simulink model "iiwa_IK_ROS"  (R2016b)
settings: Solver=FixedStepAuto  StartTime=0.0  StopTime=inf  FixedStep=0.05  RelTol=1e-3
model workspace (MAT data in the model file):
  SL_ROS_VariableLengthArrays_MaxSizes : struct (value not decoded)
libraries: robotlib x5
(part 2 of 3)

== matlab function iiwa_IK_ROS/IK/ik_solver ==
  data: js_cur_msg input; q_new output Bus: SL_Bus_iiwa_IK_ROS_sensor_msgs_JointState; E input; dQ output
% Based on transformation between /iiwa_base_link and /target_frame from tf
% as on error IK problem is solved and corresponding joint angles 
% changes is sent to arm_state topic

function [q_new, dQ]  = fcn(js_cur_msg, E)

persistent seq;
if isempty(seq)
    seq = 0;
end

q_new = js_cur_msg;
%n = q_new.Position_SL_Info.CurrentLength;

d01 = 0.36;
d23 = 0.42;
d45 = 0.4;
d67 = 0.126;

th1 = q_new.Position(1);
th2 = q_new.Position(2);
th3 = q_new.Position(3);
th4 = q_new.Position(4);
th5 = q_new.Position(5);
th6 = q_new.Position(6);
th7 = q_new.Position(7);

J7 = [ d67*(cos(th6)*(sin(th4)*(cos(th1)*sin(th3) + cos(th2)*cos(th3)*sin(th1)) + cos(th4)*sin(th1)*sin(th2)) + sin(th6)*(cos(th5)*(cos(th4)*(cos(th1)*sin(th3) + cos(th2)*cos(th3)*sin(th1)) - sin(th1)*sin(th2)*sin(th4)) + sin(th5)*(cos(th1)*cos(th3) - cos(th2)*sin(th1)*sin(th3)))) + d45*(sin(th4)*(cos(th1)*sin(th3) + cos(th2)*cos(th3)*sin(th1)) + cos(th4)*sin(th1)*sin(th2)) + d23*sin(th1)*sin(th2),                                                                                                                                                                                                                                                                                                                                                                                                                                                                                                                                                                                       -cos(th1)*(d45*(cos(th2)*cos(th4) - cos(th3)*sin(th2)*sin(th4)) - d67*(sin(th6)*(cos(th5)*(cos(th2)*sin(th4) + cos(th3)*cos(th4)*sin(th2)) - sin(th2)*sin(th3)*sin(th5)) - cos(th6)*(cos(th2)*cos(th4) - cos(th3)*sin(th2)*sin(th4))) + d23*cos(th2)),                                                                                                                                                                          cos(th2)*(d67*(cos(th6)*(sin(th4)*(cos(th1)*sin(th3) + cos(th2)*cos(th3)*sin(th1)) + cos(th4)*sin(th1)*sin(th2)) + sin(th6)*(cos(th5)*(cos(th4)*(cos(th1)*sin(th3) + cos(th2)*cos(th3)*sin(th1)) - sin(th1)*sin(th2)*sin(th4)) + sin(th5)*(cos(th1)*cos(th3) - cos(th2)*sin(th1)*sin(th3)))) + d45*(sin(th4)*(cos(th1)*sin(th3) + cos(th2)*cos(th3)*sin(th1)) + cos(th4)*sin(th1)*sin(th2)) + d23*sin(th1)*sin(th2)) - sin(th1)*sin(th2)*(d45*(cos(th2)*cos(th4) - cos(th3)*sin(th2)*sin(th4)) - d67*(sin(th6)*(cos(th5)*(cos(th2)*sin(th4) + cos(th3)*cos(th4)*sin(th2)) - sin(th2)*sin(th3)*sin(th5)) - cos(th6)*(cos(th2)*cos(th4) - cos(th3)*sin(th2)*sin(th4))) + d23*cos(th2)),                                                                                                                                                                                       sin(th2)*sin(th3)*(d67*(cos(th6)*(sin(th4)*(cos(th1)*sin(th3) + cos(th2)*cos(th3)*sin(th1)) + cos(th4)*sin(th1)*sin(th2)) + sin(th6)*(cos(th5)*(cos(th4)*(cos(th1)*sin(th3) + cos(th2)*cos(th3)*sin(th1)) - sin(th1)*sin(th2)*sin(th4)) + sin(th5)*(cos(th1)*cos(th3) - cos(th2)*sin(th1)*sin(th3)))) + d45*(sin(th4)*(cos(th1)*sin(th3) + cos(th2)*cos(th3)*sin(th1)) + cos(th4)*sin(th1)*sin(th2))) - (cos(th1)*cos(th3) - cos(th2)*sin(th1)*sin(th3))*(d45*(cos(th2)*cos(th4) - cos(th3)*sin(th2)*sin(th4)) - d67*(sin(th6)*(cos(th5)*(cos(th2)*sin(th4) + cos(th3)*cos(th4)*sin(th2)) - sin(th2)*sin(th3)*sin(th5)) - cos(th6)*(cos(th2)*cos(th4) - cos(th3)*sin(th2)*sin(th4)))),                                                                                                                                                                                                (cos(th2)*cos(th4) - cos(th3)*sin(th2)*sin(th4))*(d67*(cos(th6)*(sin(th4)*(cos(th1)*sin(th3) + cos(th2)*cos(th3)*sin(th1)) + cos(th4)*sin(th1)*sin(th2)) + sin(th6)*(cos(th5)*(cos(th4)*(cos(th1)*sin(th3) + cos(th2)*cos(th3)*sin(th1)) - sin(th1)*sin(th2)*sin(th4)) + sin(th5)*(cos(th1)*cos(th3) - cos(th2)*sin(th1)*sin(th3)))) + d45*(sin(th4)*(cos(th1)*sin(th3) + cos(th2)*cos(th3)*sin(th1)) + cos(th4)*sin(th1)*sin(th2))) - (sin(th4)*(cos(th1)*sin(th3) + cos(th2)*cos(th3)*sin(th1)) + cos(th4)*sin(th1)*sin(th2))*(d45*(cos(th2)*cos(th4) - cos(th3)*sin(th2)*sin(th4)) - d67*(sin(th6)*(cos(th5)*(cos(th2)*sin(th4) + cos(th3)*cos(th4)*sin(th2)) - sin(th2)*sin(th3)*sin(th5)) - cos(th6)*(cos(th2)*cos(th4) - cos(th3)*sin(th2)*sin(th4)))),                                                                                                                                                                                       d67*(sin(th5)*(cos(th2)*sin(th4) + cos(th3)*cos(th4)*sin(th2)) + cos(th5)*sin(th2)*sin(th3))*(cos(th6)*(sin(th4)*(cos(th1)*sin(th3) + cos(th2)*cos(th3)*sin(th1)) + cos(th4)*sin(th1)*sin(th2)) + sin(th6)*(cos(th5)*(cos(th4)*(cos(th1)*sin(th3) + cos(th2)*cos(th3)*sin(th1)) - sin(th1)*sin(th2)*sin(th4)) + sin(th5)*(cos(th1)*cos(th3) - cos(th2)*sin(th1)*sin(th3)))) - d67*(sin(th5)*(cos(th4)*(cos(th1)*sin(th3) + cos(th2)*cos(th3)*sin(th1)) - sin(th1)*sin(th2)*sin(th4)) - cos(th5)*(cos(th1)*cos(th3) - cos(th2)*sin(th1)*sin(th3)))*(sin(th6)*(cos(th5)*(cos(th2)*sin(th4) + cos(th3)*cos(th4)*sin(th2)) - sin(th2)*sin(th3)*sin(th5)) - cos(th6)*(cos(th2)*cos(th4) - cos(th3)*sin(th2)*sin(th4))),                                                                                                                                                                                                                                                                              0;...
 d67*(cos(th6)*(sin(th4)*(sin(th1)*sin(th3) - cos(th1)*cos(th2)*cos(th3)) - cos(th1)*cos(th4)*sin(th2)) + sin(th6)*(cos(th5)*(cos(th4)*(sin(th1)*sin(th3) - cos(th1)*cos(th2)*cos(th3)) + cos(th1)*sin(th2)*sin(th4)) + sin(th5)*(cos(th3)*sin(th1) + cos(th1)*cos(th2)*sin(th3)))) + d45*(sin(th4)*(sin(th1)*sin(th3) - cos(th1)*cos(th2)*cos(th3)) - cos(th1)*cos(th4)*sin(th2)) - d23*cos(th1)*sin(th2),                                                                                                                                                                                                                                                                                                                                                                                                                                                                                                                                                                                       -sin(th1)*(d45*(cos(th2)*cos(th4) - cos(th3)*sin(th2)*sin(th4)) - d67*(sin(th6)*(cos(th5)*(cos(th2)*sin(th4) + cos(th3)*cos(th4)*sin(th2)) - sin(th2)*sin(th3)*sin(th5)) - cos(th6)*(cos(th2)*cos(th4) - cos(th3)*sin(th2)*sin(th4))) + d23*cos(th2)),                                                                                                                                                                          cos(th2)*(d67*(cos(th6)*(sin(th4)*(sin(th1)*sin(th3) - cos(th1)*cos(th2)*cos(th3)) - cos(th1)*cos(th4)*sin(th2)) + sin(th6)*(cos(th5)*(cos(th4)*(sin(th1)*sin(th3) - cos(th1)*cos(th2)*cos(th3)) + cos(th1)*sin(th2)*sin(th4)) + sin(th5)*(cos(th3)*sin(th1) + cos(th1)*cos(th2)*sin(th3)))) + d45*(sin(th4)*(sin(th1)*sin(th3) - cos(th1)*cos(th2)*cos(th3)) - cos(th1)*cos(th4)*sin(th2)) - d23*cos(th1)*sin(th2)) + cos(th1)*sin(th2)*(d45*(cos(th2)*cos(th4) - cos(th3)*sin(th2)*sin(th4)) - d67*(sin(th6)*(cos(th5)*(cos(th2)*sin(th4) + cos(th3)*cos(th4)*sin(th2)) - sin(th2)*sin(th3)*sin(th5)) - cos(th6)*(cos(th2)*cos(th4) - cos(th3)*sin(th2)*sin(th4))) + d23*cos(th2)),                                                                                                                                                                                       sin(th2)*sin(th3)*(d67*(cos(th6)*(sin(th4)*(sin(th1)*sin(th3) - cos(th1)*cos(th2)*cos(th3)) - cos(th1)*cos(th4)*sin(th2)) + sin(th6)*(cos(th5)*(cos(th4)*(sin(th1)*sin(th3) - cos(th1)*cos(th2)*cos(th3)) + cos(th1)*sin(th2)*sin(th4)) + sin(th5)*(cos(th3)*sin(th1) + cos(th1)*cos(th2)*sin(th3)))) + d45*(sin(th4)*(sin(th1)*sin(th3) - cos(th1)*cos(th2)*cos(th3)) - cos(th1)*cos(th4)*sin(th2))) - (cos(th3)*sin(th1) + cos(th1)*cos(th2)*sin(th3))*(d45*(cos(th2)*cos(th4) - cos(th3)*sin(th2)*sin(th4)) - d67*(sin(th6)*(cos(th5)*(cos(th2)*sin(th4) + cos(th3)*cos(th4)*sin(th2)) - sin(th2)*sin(th3)*sin(th5)) - cos(th6)*(cos(th2)*cos(th4) - cos(th3)*sin(th2)*sin(th4)))),                                                                                                                                                                                                (d67*(cos(th6)*(sin(th4)*(sin(th1)*sin(th3) - cos(th1)*cos(th2)*cos(th3)) - cos(th1)*cos(th4)*sin(th2)) + sin(th6)*(cos(th5)*(cos(th4)*(sin(th1)*sin(th3) - cos(th1)*cos(th2)*cos(th3)) + cos(th1)*sin(th2)*sin(th4)) + sin(th5)*(cos(th3)*sin(th1) + cos(th1)*cos(th2)*sin(th3)))) + d45*(sin(th4)*(sin(th1)*sin(th3) - cos(th1)*cos(th2)*cos(th3)) - cos(th1)*cos(th4)*sin(th2)))*(cos(th2)*cos(th4) - cos(th3)*sin(th2)*sin(th4)) - (sin(th4)*(sin(th1)*sin(th3) - cos(th1)*cos(th2)*cos(th3)) - cos(th1)*cos(th4)*sin(th2))*(d45*(cos(th2)*cos(th4) - cos(th3)*sin(th2)*sin(th4)) - d67*(sin(th6)*(cos(th5)*(cos(th2)*sin(th4) + cos(th3)*cos(th4)*sin(th2)) - sin(th2)*sin(th3)*sin(th5)) - cos(th6)*(cos(th2)*cos(th4) - cos(th3)*sin(th2)*sin(th4)))),                                                                                                                                                                                       d67*(sin(th5)*(cos(th2)*sin(th4) + cos(th3)*cos(th4)*sin(th2)) + cos(th5)*sin(th2)*sin(th3))*(cos(th6)*(sin(th4)*(sin(th1)*sin(th3) - cos(th1)*cos(th2)*cos(th3)) - cos(th1)*cos(th4)*sin(th2)) + sin(th6)*(cos(th5)*(cos(th4)*(sin(th1)*sin(th3) - cos(th1)*cos(th2)*cos(th3)) + cos(th1)*sin(th2)*sin(th4)) + sin(th5)*(cos(th3)*sin(th1) + cos(th1)*cos(th2)*sin(th3)))) - d67*(sin(th5)*(cos(th4)*(sin(th1)*sin(th3) - cos(th1)*cos(th2)*cos(th3)) + cos(th1)*sin(th2)*sin(th4)) - cos(th5)*(cos(th3)*sin(th1) + cos(th1)*cos(th2)*sin(th3)))*(sin(th6)*(cos(th5)*(cos(th2)*sin(th4) + cos(th3)*cos(th4)*sin(th2)) - sin(th2)*sin(th3)*sin(th5)) - cos(th6)*(cos(th2)*cos(th4) - cos(th3)*sin(th2)*sin(th4))),                                                                                                                                                                                                                                                                              0;...
                                                                                                                                                                                                                                                                                                                                                                                                         0, cos(th1)*(d67*(cos(th6)*(sin(th4)*(sin(th1)*sin(th3) - cos(th1)*cos(th2)*cos(th3)) - cos(th1)*cos(th4)*sin(th2)) + sin(th6)*(cos(th5)*(cos(th4)*(sin(th1)*sin(th3) - cos(th1)*cos(th2)*cos(th3)) + cos(th1)*sin(th2)*sin(th4)) + sin(th5)*(cos(th3)*sin(th1) + cos(th1)*cos(th2)*sin(th3)))) + d45*(sin(th4)*(sin(th1)*sin(th3) - cos(th1)*cos(th2)*cos(th3)) - cos(th1)*cos(th4)*sin(th2)) - d23*cos(th1)*sin(th2)) - sin(th1)*(d67*(cos(th6)*(sin(th4)*(cos(th1)*sin(th3) + cos(th2)*cos(th3)*sin(th1)) + cos(th4)*sin(th1)*sin(th2)) + sin(th6)*(cos(th5)*(cos(th4)*(cos(th1)*sin(th3) + cos(th2)*cos(th3)*sin(th1)) - sin(th1)*sin(th2)*sin(th4)) + sin(th5)*(cos(th1)*cos(th3) - cos(th2)*sin(th1)*sin(th3)))) + d45*(sin(th4)*(cos(th1)*sin(th3) + cos(th2)*cos(th3)*sin(th1)) + cos(th4)*sin(th1)*sin(th2)) + d23*sin(th1)*sin(th2)), sin(th1)*sin(th2)*(d67*(cos(th6)*(sin(th4)*(sin(th1)*sin(th3) - cos(th1)*cos(th2)*cos(th3)) - cos(th1)*cos(th4)*sin(th2)) + sin(th6)*(cos(th5)*(cos(th4)*(sin(th1)*sin(th3) - cos(th1)*cos(th2)*cos(th3)) + cos(th1)*sin(th2)*sin(th4)) + sin(th5)*(cos(th3)*sin(th1) + cos(th1)*cos(th2)*sin(th3)))) + d45*(sin(th4)*(sin(th1)*sin(th3) - cos(th1)*cos(th2)*cos(th3)) - cos(th1)*cos(th4)*sin(th2)) - d23*cos(th1)*sin(th2)) + cos(th1)*sin(th2)*(d67*(cos(th6)*(sin(th4)*(cos(th1)*sin(th3) + cos(th2)*cos(th3)*sin(th1)) + cos(th4)*sin(th1)*sin(th2)) + sin(th6)*(cos(th5)*(cos(th4)*(cos(th1)*sin(th3) + cos(th2)*cos(th3)*sin(th1)) - sin(th1)*sin(th2)*sin(th4)) + sin(th5)*(cos(th1)*cos(th3) - cos(th2)*sin(th1)*sin(th3)))) + d45*(sin(th4)*(cos(th1)*sin(th3) + cos(th2)*cos(th3)*sin(th1)) + cos(th4)*sin(th1)*sin(th2)) + d23*sin(th1)*sin(th2)), (d67*(cos(th6)*(sin(th4)*(sin(th1)*sin(th3) - cos(th1)*cos(th2)*cos(th3)) - cos(th1)*cos(th4)*sin(th2)) + sin(th6)*(cos(th5)*(cos(th4)*(sin(th1)*sin(th3) - cos(th1)*cos(th2)*cos(th3)) + cos(th1)*sin(th2)*sin(th4)) + sin(th5)*(cos(th3)*sin(th1) + cos(th1)*cos(th2)*sin(th3)))) + d45*(sin(th4)*(sin(th1)*sin(th3) - cos(th1)*cos(th2)*cos(th3)) - cos(th1)*cos(th4)*sin(th2)))*(cos(th1)*cos(th3) - cos(th2)*sin(th1)*sin(th3)) - (cos(th3)*sin(th1) + cos(th1)*cos(th2)*sin(th3))*(d67*(cos(th6)*(sin(th4)*(cos(th1)*sin(th3) + cos(th2)*cos(th3)*sin(th1)) + cos(th4)*sin(th1)*sin(th2)) + sin(th6)*(cos(th5)*(cos(th4)*(cos(th1)*sin(th3) + cos(th2)*cos(th3)*sin(th1)) - sin(th1)*sin(th2)*sin(th4)) + sin(th5)*(cos(th1)*cos(th3) - cos(th2)*sin(th1)*sin(th3)))) + d45*(sin(th4)*(cos(th1)*sin(th3) + cos(th2)*cos(th3)*sin(th1)) + cos(th4)*sin(th1)*sin(th2))), (sin(th4)*(cos(th1)*sin(th3) + cos(th2)*cos(th3)*sin(th1)) + cos(th4)*sin(th1)*sin(th2))*(d67*(cos(th6)*(sin(th4)*(sin(th1)*sin(th3) - cos(th1)*cos(th2)*cos(th3)) - cos(th1)*cos(th4)*sin(th2)) + sin(th6)*(cos(th5)*(cos(th4)*(sin(th1)*sin(th3) - cos(th1)*cos(th2)*cos(th3)) + cos(th1)*sin(th2)*sin(th4)) + sin(th5)*(cos(th3)*sin(th1) + cos(th1)*cos(th2)*sin(th3)))) + d45*(sin(th4)*(sin(th1)*sin(th3) - cos(th1)*cos(th2)*cos(th3)) - cos(th1)*cos(th4)*sin(th2))) - (sin(th4)*(sin(th1)*sin(th3) - cos(th1)*cos(th2)*cos(th3)) - cos(th1)*cos(th4)*sin(th2))*(d67*(cos(th6)*(sin(th4)*(cos(th1)*sin(th3) + cos(th2)*cos(th3)*sin(th1)) + cos(th4)*sin(th1)*sin(th2)) + sin(th6)*(cos(th5)*(cos(th4)*(cos(th1)*sin(th3) + cos(th2)*cos(th3)*sin(th1)) - sin(th1)*sin(th2)*sin(th4)) + sin(th5)*(cos(th1)*cos(th3) - cos(th2)*sin(th1)*sin(th3)))) + d45*(sin(th4)*(cos(th1)*sin(th3) + cos(th2)*cos(th3)*sin(th1)) + cos(th4)*sin(th1)*sin(th2))), d67*(sin(th5)*(cos(th4)*(sin(th1)*sin(th3) - cos(th1)*cos(th2)*cos(th3)) + cos(th1)*sin(th2)*sin(th4)) - cos(th5)*(cos(th3)*sin(th1) + cos(th1)*cos(th2)*sin(th3)))*(cos(th6)*(sin(th4)*(cos(th1)*sin(th3) + cos(th2)*cos(th3)*sin(th1)) + cos(th4)*sin(th1)*sin(th2)) + sin(th6)*(cos(th5)*(cos(th4)*(cos(th1)*sin(th3) + cos(th2)*cos(th3)*sin(th1)) - sin(th1)*sin(th2)*sin(th4)) + sin(th5)*(cos(th1)*cos(th3) - cos(th2)*sin(th1)*sin(th3)))) - d67*(cos(th6)*(sin(th4)*(sin(th1)*sin(th3) - cos(th1)*cos(th2)*cos(th3)) - cos(th1)*cos(th4)*sin(th2)) + sin(th6)*(cos(th5)*(cos(th4)*(sin(th1)*sin(th3) - cos(th1)*cos(th2)*cos(th3)) + cos(th1)*sin(th2)*sin(th4)) + sin(th5)*(cos(th3)*sin(th1) + cos(th1)*cos(th2)*sin(th3))))*(sin(th5)*(cos(th4)*(cos(th1)*sin(th3) + cos(th2)*cos(th3)*sin(th1)) - sin(th1)*sin(th2)*sin(th4)) - cos(th5)*(cos(th1)*cos(th3) - cos(th2)*sin(th1)*sin(th3))),                                                                                                                                                                                                                                                                              0;...
                                                                                                                                                                                                                                                                                                                                                                                                         0,                                                                                                                                                                                                                                                                                                                                                                                                                                                                                                                                                                                                                                                                                                                                                                                                                                    sin(th1),                                                                                                                                                                                                                                                                                                                                                                                                                                                                                                                                                                                                                                                                                                                                                                                                                                            -cos(th1)*sin(th2),                                                                                                                                                                                                                                                                                                                                                                                                                                                                                                                                                                                                                                                                                                                                                                                                                              cos(th3)*sin(th1) + cos(th1)*cos(th2)*sin(th3),                                                                                                                                                                                                                                                                                                                                                                                                                                                                                                                                                                                                                                                                                                                                                                                                                                                                      sin(th4)*(sin(th1)*sin(th3) - cos(th1)*cos(th2)*cos(th3)) - cos(th1)*cos(th4)*sin(th2),                                                                                                                                                                                                                                                                                                                                                                                                                                                                                                                                                                                                                                                                                                                                           cos(th5)*(cos(th3)*sin(th1) + cos(th1)*cos(th2)*sin(th3)) - sin(th5)*(cos(th4)*(sin(th1)*sin(th3) - cos(th1)*cos(th2)*cos(th3)) + cos(th1)*sin(th2)*sin(th4)),   cos(th6)*(sin(th4)*(sin(th1)*sin(th3) - cos(th1)*cos(th2)*cos(th3)) - cos(th1)*cos(th4)*sin(th2)) + sin(th6)*(cos(th5)*(cos(th4)*(sin(th1)*sin(th3) - cos(th1)*cos(th2)*cos(th3)) + cos(th1)*sin(th2)*sin(th4)) + sin(th5)*(cos(th3)*sin(th1) + cos(th1)*cos(th2)*sin(th3)));...
                                                                                                                                                                                                                                                                                                                                                                                                         0,                                                                                                                                                                                                                                                                                                                                                                                                                                                                                                                                                                                                                                                                                                                                                                                                                                   -cos(th1),                                                                                                                                                                                                                                                                                                                                                                                                                                                                                                                                                                                                                                                                                                                                                                                                                                            -sin(th1)*sin(th2),                                                                                                                                                                                                                                                                                                                                                                                                                                                                                                                                                                                                                                                                                                                                                                                                                              cos(th2)*sin(th1)*sin(th3) - cos(th1)*cos(th3),                                                                                                                                                                                                                                                                                                                                                                                                                                                                                                                                                                                                                                                                                                                                                                                                                                                                    - sin(th4)*(cos(th1)*sin(th3) + cos(th2)*cos(th3)*sin(th1)) - cos(th4)*sin(th1)*sin(th2),                                                                                                                                                                                                                                                                                                                                                                                                                                                                                                                                                                                                                                                                                                                                           sin(th5)*(cos(th4)*(cos(th1)*sin(th3) + cos(th2)*cos(th3)*sin(th1)) - sin(th1)*sin(th2)*sin(th4)) - cos(th5)*(cos(th1)*cos(th3) - cos(th2)*sin(th1)*sin(th3)), - cos(th6)*(sin(th4)*(cos(th1)*sin(th3) + cos(th2)*cos(th3)*sin(th1)) + cos(th4)*sin(th1)*sin(th2)) - sin(th6)*(cos(th5)*(cos(th4)*(cos(th1)*sin(th3) + cos(th2)*cos(th3)*sin(th1)) - sin(th1)*sin(th2)*sin(th4)) + sin(th5)*(cos(th1)*cos(th3) - cos(th2)*sin(th1)*sin(th3)));...
                                                                                                                                                                                                                                                                                                                                                                                                         1,                                                                                                                                                                                                                                                                                                                                                                                                                                                                                                                                                                                                                                                                                                                                                                                                                                           0,                                                                                                                                                                                                                                                                                                                                                                                                                                                                                                                                                                                                                                                                                                                                                                                                                                                      cos(th2),                                                                                                                                                                                                                                                                                                                                                                                                                                                                                                                                                                                                                                                                                                                                                                                                                                                           sin(th2)*sin(th3),                                                                                                                                                                                                                                                                                                                                                                                                                                                                                                                                                                                                                                                                                                                                                                                                                                                                                                              cos(th2)*cos(th4) - cos(th3)*sin(th2)*sin(th4),                                                                                                                                                                                                                                                                                                                                                                                                                                                                                                                                                                                                                                                                                                                                                                                                                  sin(th5)*(cos(th2)*sin(th4) + cos(th3)*cos(th4)*sin(th2)) + cos(th5)*sin(th2)*sin(th3),                                                                                                                  cos(th6)*(cos(th2)*cos(th4) - cos(th3)*sin(th2)*sin(th4)) - sin(th6)*(cos(th5)*(cos(th2)*sin(th4) + cos(th3)*cos(th4)*sin(th2)) - sin(th2)*sin(th3)*sin(th5))];
%%%%%%%%%%%%%%%%%%%%%%%%%%%%%%%%%%%%%%%%%%%%%

J7t = [                                                                                                                                                                                                                                                                                                                                                    d67*(cos(th6)*(sin(th4)*(cos(th1)*sin(th3) + cos(th2)*cos(th3)*sin(th1)) + cos(th4)*sin(th1)*sin(th2)) + sin(th6)*(cos(th5)*(cos(th4)*(cos(th1)*sin(th3) + cos(th2)*cos(th3)*sin(th1)) - sin(th1)*sin(th2)*sin(th4)) + sin(th5)*(cos(th1)*cos(th3) - cos(th2)*sin(th1)*sin(th3)))) + d45*(sin(th4)*(cos(th1)*sin(th3) + cos(th2)*cos(th3)*sin(th1)) + cos(th4)*sin(th1)*sin(th2)) + d23*sin(th1)*sin(th2),                                                                                                                                                                                                                                                                                                                                                    d67*(cos(th6)*(sin(th4)*(sin(th1)*sin(th3) - cos(th1)*cos(th2)*cos(th3)) - cos(th1)*cos(th4)*sin(th2)) + sin(th6)*(cos(th5)*(cos(th4)*(sin(th1)*sin(th3) - cos(th1)*cos(th2)*cos(th3)) + cos(th1)*sin(th2)*sin(th4)) + sin(th5)*(cos(th3)*sin(th1) + cos(th1)*cos(th2)*sin(th3)))) + d45*(sin(th4)*(sin(th1)*sin(th3) - cos(th1)*cos(th2)*cos(th3)) - cos(th1)*cos(th4)*sin(th2)) - d23*cos(th1)*sin(th2),                                                                                                                                                                                                                                                                                                                                                                                                                                                                                                                                                                                                                                                                                                                                                                                                                                                                                                                                                           0,                                                                                                                                                                                                                                                                            0,                                                                                                                                                                                                                                                                              0,                                                                                                                                                             1;...
                                                                                                                                                                                                                                                                                                                                                                                                                                                                                                        -cos(th1)*(d45*(cos(th2)*cos(th4) - cos(th3)*sin(th2)*sin(th4)) - d67*(sin(th6)*(cos(th5)*(cos(th2)*sin(th4) + cos(th3)*cos(th4)*sin(th2)) - sin(th2)*sin(th3)*sin(th5)) - cos(th6)*(cos(th2)*cos(th4) - cos(th3)*sin(th2)*sin(th4))) + d23*cos(th2)),                                                                                                                                                                                                                                                                                                                                                                                                                                                                                                        -sin(th1)*(d45*(cos(th2)*cos(th4) - cos(th3)*sin(th2)*sin(th4)) - d67*(sin(th6)*(cos(th5)*(cos(th2)*sin(th4) + cos(th3)*cos(th4)*sin(th2)) - sin(th2)*sin(th3)*sin(th5)) - cos(th6)*(cos(th2)*cos(th4) - cos(th3)*sin(th2)*sin(th4))) + d23*cos(th2)),                                                                                                                 cos(th1)*(d67*(cos(th6)*(sin(th4)*(sin(th1)*sin(th3) - cos(th1)*cos(th2)*cos(th3)) - cos(th1)*cos(th4)*sin(th2)) + sin(th6)*(cos(th5)*(cos(th4)*(sin(th1)*sin(th3) - cos(th1)*cos(th2)*cos(th3)) + cos(th1)*sin(th2)*sin(th4)) + sin(th5)*(cos(th3)*sin(th1) + cos(th1)*cos(th2)*sin(th3)))) + d45*(sin(th4)*(sin(th1)*sin(th3) - cos(th1)*cos(th2)*cos(th3)) - cos(th1)*cos(th4)*sin(th2)) - d23*cos(th1)*sin(th2)) - sin(th1)*(d67*(cos(th6)*(sin(th4)*(cos(th1)*sin(th3) + cos(th2)*cos(th3)*sin(th1)) + cos(th4)*sin(th1)*sin(th2)) + sin(th6)*(cos(th5)*(cos(th4)*(cos(th1)*sin(th3) + cos(th2)*cos(th3)*sin(th1)) - sin(th1)*sin(th2)*sin(th4)) + sin(th5)*(cos(th1)*cos(th3) - cos(th2)*sin(th1)*sin(th3)))) + d45*(sin(th4)*(cos(th1)*sin(th3) + cos(th2)*cos(th3)*sin(th1)) + cos(th4)*sin(th1)*sin(th2)) + d23*sin(th1)*sin(th2)),                                                                                                                                                                                                                                                                     sin(th1),                                                                                                                                                                                                                                                                      -cos(th1),                                                                                                                                                             0;...
                                                                         cos(th2)*(d67*(cos(th6)*(sin(th4)*(cos(th1)*sin(th3) + cos(th2)*cos(th3)*sin(th1)) + cos(th4)*sin(th1)*sin(th2)) + sin(th6)*(cos(th5)*(cos(th4)*(cos(th1)*sin(th3) + cos(th2)*cos(th3)*sin(th1)) - sin(th1)*sin(th2)*sin(th4)) + sin(th5)*(cos(th1)*cos(th3) - cos(th2)*sin(th1)*sin(th3)))) + d45*(sin(th4)*(cos(th1)*sin(th3) + cos(th2)*cos(th3)*sin(th1)) + cos(th4)*sin(th1)*sin(th2)) + d23*sin(th1)*sin(th2)) - sin(th1)*sin(th2)*(d45*(cos(th2)*cos(th4) - cos(th3)*sin(th2)*sin(th4)) - d67*(sin(th6)*(cos(th5)*(cos(th2)*sin(th4) + cos(th3)*cos(th4)*sin(th2)) - sin(th2)*sin(th3)*sin(th5)) - cos(th6)*(cos(th2)*cos(th4) - cos(th3)*sin(th2)*sin(th4))) + d23*cos(th2)),                                                                         cos(th2)*(d67*(cos(th6)*(sin(th4)*(sin(th1)*sin(th3) - cos(th1)*cos(th2)*cos(th3)) - cos(th1)*cos(th4)*sin(th2)) + sin(th6)*(cos(th5)*(cos(th4)*(sin(th1)*sin(th3) - cos(th1)*cos(th2)*cos(th3)) + cos(th1)*sin(th2)*sin(th4)) + sin(th5)*(cos(th3)*sin(th1) + cos(th1)*cos(th2)*sin(th3)))) + d45*(sin(th4)*(sin(th1)*sin(th3) - cos(th1)*cos(th2)*cos(th3)) - cos(th1)*cos(th4)*sin(th2)) - d23*cos(th1)*sin(th2)) + cos(th1)*sin(th2)*(d45*(cos(th2)*cos(th4) - cos(th3)*sin(th2)*sin(th4)) - d67*(sin(th6)*(cos(th5)*(cos(th2)*sin(th4) + cos(th3)*cos(th4)*sin(th2)) - sin(th2)*sin(th3)*sin(th5)) - cos(th6)*(cos(th2)*cos(th4) - cos(th3)*sin(th2)*sin(th4))) + d23*cos(th2)),                                                                                               sin(th1)*sin(th2)*(d67*(cos(th6)*(sin(th4)*(sin(th1)*sin(th3) - cos(th1)*cos(th2)*cos(th3)) - cos(th1)*cos(th4)*sin(th2)) + sin(th6)*(cos(th5)*(cos(th4)*(sin(th1)*sin(th3) - cos(th1)*cos(th2)*cos(th3)) + cos(th1)*sin(th2)*sin(th4)) + sin(th5)*(cos(th3)*sin(th1) + cos(th1)*cos(th2)*sin(th3)))) + d45*(sin(th4)*(sin(th1)*sin(th3) - cos(th1)*cos(th2)*cos(th3)) - cos(th1)*cos(th4)*sin(th2)) - d23*cos(th1)*sin(th2)) + cos(th1)*sin(th2)*(d67*(cos(th6)*(sin(th4)*(cos(th1)*sin(th3) + cos(th2)*cos(th3)*sin(th1)) + cos(th4)*sin(th1)*sin(th2)) + sin(th6)*(cos(th5)*(cos(th4)*(cos(th1)*sin(th3) + cos(th2)*cos(th3)*sin(th1)) - sin(th1)*sin(th2)*sin(th4)) + sin(th5)*(cos(th1)*cos(th3) - cos(th2)*sin(th1)*sin(th3)))) + d45*(sin(th4)*(cos(th1)*sin(th3) + cos(th2)*cos(th3)*sin(th1)) + cos(th4)*sin(th1)*sin(th2)) + d23*sin(th1)*sin(th2)),                                                                                                                                                                                                                                                           -cos(th1)*sin(th2),                                                                                                                                                                                                                                                             -sin(th1)*sin(th2),                                                                                                                                                      cos(th2);...
                                                                        sin(th2)*sin(th3)*(d67*(cos(th6)*(sin(th4)*(cos(th1)*sin(th3) + cos(th2)*cos(th3)*sin(th1)) + cos(th4)*sin(th1)*sin(th2)) + sin(th6)*(cos(th5)*(cos(th4)*(cos(th1)*sin(th3) + cos(th2)*cos(th3)*sin(th1)) - sin(th1)*sin(th2)*sin(th4)) + sin(th5)*(cos(th1)*cos(th3) - cos(th2)*sin(th1)*sin(th3)))) + d45*(sin(th4)*(cos(th1)*sin(th3) + cos(th2)*cos(th3)*sin(th1)) + cos(th4)*sin(th1)*sin(th2))) - (cos(th1)*cos(th3) - cos(th2)*sin(th1)*sin(th3))*(d45*(cos(th2)*cos(th4) - cos(th3)*sin(th2)*sin(th4)) - d67*(sin(th6)*(cos(th5)*(cos(th2)*sin(th4) + cos(th3)*cos(th4)*sin(th2)) - sin(th2)*sin(th3)*sin(th5)) - cos(th6)*(cos(th2)*cos(th4) - cos(th3)*sin(th2)*sin(th4)))),                                                                        sin(th2)*sin(th3)*(d67*(cos(th6)*(sin(th4)*(sin(th1)*sin(th3) - cos(th1)*cos(th2)*cos(th3)) - cos(th1)*cos(th4)*sin(th2)) + sin(th6)*(cos(th5)*(cos(th4)*(sin(th1)*sin(th3) - cos(th1)*cos(th2)*cos(th3)) + cos(th1)*sin(th2)*sin(th4)) + sin(th5)*(cos(th3)*sin(th1) + cos(th1)*cos(th2)*sin(th3)))) + d45*(sin(th4)*(sin(th1)*sin(th3) - cos(th1)*cos(th2)*cos(th3)) - cos(th1)*cos(th4)*sin(th2))) - (cos(th3)*sin(th1) + cos(th1)*cos(th2)*sin(th3))*(d45*(cos(th2)*cos(th4) - cos(th3)*sin(th2)*sin(th4)) - d67*(sin(th6)*(cos(th5)*(cos(th2)*sin(th4) + cos(th3)*cos(th4)*sin(th2)) - sin(th2)*sin(th3)*sin(th5)) - cos(th6)*(cos(th2)*cos(th4) - cos(th3)*sin(th2)*sin(th4)))),                                                                                 (d67*(cos(th6)*(sin(th4)*(sin(th1)*sin(th3) - cos(th1)*cos(th2)*cos(th3)) - cos(th1)*cos(th4)*sin(th2)) + sin(th6)*(cos(th5)*(cos(th4)*(sin(th1)*sin(th3) - cos(th1)*cos(th2)*cos(th3)) + cos(th1)*sin(th2)*sin(th4)) + sin(th5)*(cos(th3)*sin(th1) + cos(th1)*cos(th2)*sin(th3)))) + d45*(sin(th4)*(sin(th1)*sin(th3) - cos(th1)*cos(th2)*cos(th3)) - cos(th1)*cos(th4)*sin(th2)))*(cos(th1)*cos(th3) - cos(th2)*sin(th1)*sin(th3)) - (cos(th3)*sin(th1) + cos(th1)*cos(th2)*sin(th3))*(d67*(cos(th6)*(sin(th4)*(cos(th1)*sin(th3) + cos(th2)*cos(th3)*sin(th1)) + cos(th4)*sin(th1)*sin(th2)) + sin(th6)*(cos(th5)*(cos(th4)*(cos(th1)*sin(th3) + cos(th2)*cos(th3)*sin(th1)) - sin(th1)*sin(th2)*sin(th4)) + sin(th5)*(cos(th1)*cos(th3) - cos(th2)*sin(th1)*sin(th3)))) + d45*(sin(th4)*(cos(th1)*sin(th3) + cos(th2)*cos(th3)*sin(th1)) + cos(th4)*sin(th1)*sin(th2))),                                                                                                                                                                                                                               cos(th3)*sin(th1) + cos(th1)*cos(th2)*sin(th3),                                                                                                                                                                                                                                 cos(th2)*sin(th1)*sin(th3) - cos(th1)*cos(th3),                                                                                                                                             sin(th2)*sin(th3);...
 (cos(th2)*cos(th4) - cos(th3)*sin(th2)*sin(th4))*(d67*(cos(th6)*(sin(th4)*(cos(th1)*sin(th3) + cos(th2)*cos(th3)*sin(th1)) + cos(th4)*sin(th1)*sin(th2)) + sin(th6)*(cos(th5)*(cos(th4)*(cos(th1)*sin(th3) + cos(th2)*cos(th3)*sin(th1)) - sin(th1)*sin(th2)*sin(th4)) + sin(th5)*(cos(th1)*cos(th3) - cos(th2)*sin(th1)*sin(th3)))) + d45*(sin(th4)*(cos(th1)*sin(th3) + cos(th2)*cos(th3)*sin(th1)) + cos(th4)*sin(th1)*sin(th2))) - (sin(th4)*(cos(th1)*sin(th3) + cos(th2)*cos(th3)*sin(th1)) + cos(th4)*sin(th1)*sin(th2))*(d45*(cos(th2)*cos(th4) - cos(th3)*sin(th2)*sin(th4)) - d67*(sin(th6)*(cos(th5)*(cos(th2)*sin(th4) + cos(th3)*cos(th4)*sin(th2)) - sin(th2)*sin(th3)*sin(th5)) - cos(th6)*(cos(th2)*cos(th4) - cos(th3)*sin(th2)*sin(th4)))), (d67*(cos(th6)*(sin(th4)*(sin(th1)*sin(th3) - cos(th1)*cos(th2)*cos(th3)) - cos(th1)*cos(th4)*sin(th2)) + sin(th6)*(cos(th5)*(cos(th4)*(sin(th1)*sin(th3) - cos(th1)*cos(th2)*cos(th3)) + cos(th1)*sin(th2)*sin(th4)) + sin(th5)*(cos(th3)*sin(th1) + cos(th1)*cos(th2)*sin(th3)))) + d45*(sin(th4)*(sin(th1)*sin(th3) - cos(th1)*cos(th2)*cos(th3)) - cos(th1)*cos(th4)*sin(th2)))*(cos(th2)*cos(th4) - cos(th3)*sin(th2)*sin(th4)) - (sin(th4)*(sin(th1)*sin(th3) - cos(th1)*cos(th2)*cos(th3)) - cos(th1)*cos(th4)*sin(th2))*(d45*(cos(th2)*cos(th4) - cos(th3)*sin(th2)*sin(th4)) - d67*(sin(th6)*(cos(th5)*(cos(th2)*sin(th4) + cos(th3)*cos(th4)*sin(th2)) - sin(th2)*sin(th3)*sin(th5)) - cos(th6)*(cos(th2)*cos(th4) - cos(th3)*sin(th2)*sin(th4)))), (sin(th4)*(cos(th1)*sin(th3) + cos(th2)*cos(th3)*sin(th1)) + cos(th4)*sin(th1)*sin(th2))*(d67*(cos(th6)*(sin(th4)*(sin(th1)*sin(th3) - cos(th1)*cos(th2)*cos(th3)) - cos(th1)*cos(th4)*sin(th2)) + sin(th6)*(cos(th5)*(cos(th4)*(sin(th1)*sin(th3) - cos(th1)*cos(th2)*cos(th3)) + cos(th1)*sin(th2)*sin(th4)) + sin(th5)*(cos(th3)*sin(th1) + cos(th1)*cos(th2)*sin(th3)))) + d45*(sin(th4)*(sin(th1)*sin(th3) - cos(th1)*cos(th2)*cos(th3)) - cos(th1)*cos(th4)*sin(th2))) - (sin(th4)*(sin(th1)*sin(th3) - cos(th1)*cos(th2)*cos(th3)) - cos(th1)*cos(th4)*sin(th2))*(d67*(cos(th6)*(sin(th4)*(cos(th1)*sin(th3) + cos(th2)*cos(th3)*sin(th1)) + cos(th4)*sin(th1)*sin(th2)) + sin(th6)*(cos(th5)*(cos(th4)*(cos(th1)*sin(th3) + cos(th2)*cos(th3)*sin(th1)) - sin(th1)*sin(th2)*sin(th4)) + sin(th5)*(cos(th1)*cos(th3) - cos(th2)*sin(th1)*sin(th3)))) + d45*(sin(th4)*(cos(th1)*sin(th3) + cos(th2)*cos(th3)*sin(th1)) + cos(th4)*sin(th1)*sin(th2))),                                                                                                                                                                                       sin(th4)*(sin(th1)*sin(th3) - cos(th1)*cos(th2)*cos(th3)) - cos(th1)*cos(th4)*sin(th2),                                                                                                                                                                                       - sin(th4)*(cos(th1)*sin(th3) + cos(th2)*cos(th3)*sin(th1)) - cos(th4)*sin(th1)*sin(th2),                                                                                                                cos(th2)*cos(th4) - cos(th3)*sin(th2)*sin(th4);...
                                            d67*(sin(th5)*(cos(th2)*sin(th4) + cos(th3)*cos(th4)*sin(th2)) + cos(th5)*sin(th2)*sin(th3))*(cos(th6)*(sin(th4)*(cos(th1)*sin(th3) + cos(th2)*cos(th3)*sin(th1)) + cos(th4)*sin(th1)*sin(th2)) + sin(th6)*(cos(th5)*(cos(th4)*(cos(th1)*sin(th3) + cos(th2)*cos(th3)*sin(th1)) - sin(th1)*sin(th2)*sin(th4)) + sin(th5)*(cos(th1)*cos(th3) - cos(th2)*sin(th1)*sin(th3)))) - d67*(sin(th5)*(cos(th4)*(cos(th1)*sin(th3) + cos(th2)*cos(th3)*sin(th1)) - sin(th1)*sin(th2)*sin(th4)) - cos(th5)*(cos(th1)*cos(th3) - cos(th2)*sin(th1)*sin(th3)))*(sin(th6)*(cos(th5)*(cos(th2)*sin(th4) + cos(th3)*cos(th4)*sin(th2)) - sin(th2)*sin(th3)*sin(th5)) - cos(th6)*(cos(th2)*cos(th4) - cos(th3)*sin(th2)*sin(th4))),                                            d67*(sin(th5)*(cos(th2)*sin(th4) + cos(th3)*cos(th4)*sin(th2)) + cos(th5)*sin(th2)*sin(th3))*(cos(th6)*(sin(th4)*(sin(th1)*sin(th3) - cos(th1)*cos(th2)*cos(th3)) - cos(th1)*cos(th4)*sin(th2)) + sin(th6)*(cos(th5)*(cos(th4)*(sin(th1)*sin(th3) - cos(th1)*cos(th2)*cos(th3)) + cos(th1)*sin(th2)*sin(th4)) + sin(th5)*(cos(th3)*sin(th1) + cos(th1)*cos(th2)*sin(th3)))) - d67*(sin(th5)*(cos(th4)*(sin(th1)*sin(th3) - cos(th1)*cos(th2)*cos(th3)) + cos(th1)*sin(th2)*sin(th4)) - cos(th5)*(cos(th3)*sin(th1) + cos(th1)*cos(th2)*sin(th3)))*(sin(th6)*(cos(th5)*(cos(th2)*sin(th4) + cos(th3)*cos(th4)*sin(th2)) - sin(th2)*sin(th3)*sin(th5)) - cos(th6)*(cos(th2)*cos(th4) - cos(th3)*sin(th2)*sin(th4))),                                                     d67*(sin(th5)*(cos(th4)*(sin(th1)*sin(th3) - cos(th1)*cos(th2)*cos(th3)) + cos(th1)*sin(th2)*sin(th4)) - cos(th5)*(cos(th3)*sin(th1) + cos(th1)*cos(th2)*sin(th3)))*(cos(th6)*(sin(th4)*(cos(th1)*sin(th3) + cos(th2)*cos(th3)*sin(th1)) + cos(th4)*sin(th1)*sin(th2)) + sin(th6)*(cos(th5)*(cos(th4)*(cos(th1)*sin(th3) + cos(th2)*cos(th3)*sin(th1)) - sin(th1)*sin(th2)*sin(th4)) + sin(th5)*(cos(th1)*cos(th3) - cos(th2)*sin(th1)*sin(th3)))) - d67*(cos(th6)*(sin(th4)*(sin(th1)*sin(th3) - cos(th1)*cos(th2)*cos(th3)) - cos(th1)*cos(th4)*sin(th2)) + sin(th6)*(cos(th5)*(cos(th4)*(sin(th1)*sin(th3) - cos(th1)*cos(th2)*cos(th3)) + cos(th1)*sin(th2)*sin(th4)) + sin(th5)*(cos(th3)*sin(th1) + cos(th1)*cos(th2)*sin(th3))))*(sin(th5)*(cos(th4)*(cos(th1)*sin(th3) + cos(th2)*cos(th3)*sin(th1)) - sin(th1)*sin(th2)*sin(th4)) - cos(th5)*(cos(th1)*cos(th3) - cos(th2)*sin(th1)*sin(th3))),                                                                                                                cos(th5)*(cos(th3)*sin(th1) + cos(th1)*cos(th2)*sin(th3)) - sin(th5)*(cos(th4)*(sin(th1)*sin(th3) - cos(th1)*cos(th2)*cos(th3)) + cos(th1)*sin(th2)*sin(th4)),                                                                                                                  sin(th5)*(cos(th4)*(cos(th1)*sin(th3) + cos(th2)*cos(th3)*sin(th1)) - sin(th1)*sin(th2)*sin(th4)) - cos(th5)*(cos(th1)*cos(th3) - cos(th2)*sin(th1)*sin(th3)),                                                                        sin(th5)*(cos(th2)*sin(th4) + cos(th3)*cos(th4)*sin(th2)) + cos(th5)*sin(th2)*sin(th3);...
                                                                                                                                                                                                                                                                                                                                                                                                                                                                                                                                                                                                                                                                                                                                                            0,                                                                                                                                                                                                                                                                                                                                                                                                                                                                                                                                                                                                                                                                                                                                                            0,                                                                                                                                                                                                                                                                                                                                                                                                                                                                                                                                                                                                                                                                                                                                                                                                                                                                                                                                                           0, cos(th6)*(sin(th4)*(sin(th1)*sin(th3) - cos(th1)*cos(th2)*cos(th3)) - cos(th1)*cos(th4)*sin(th2)) + sin(th6)*(cos(th5)*(cos(th4)*(sin(th1)*sin(th3) - cos(th1)*cos(th2)*cos(th3)) + cos(th1)*sin(th2)*sin(th4)) + sin(th5)*(cos(th3)*sin(th1) + cos(th1)*cos(th2)*sin(th3))), - cos(th6)*(sin(th4)*(cos(th1)*sin(th3) + cos(th2)*cos(th3)*sin(th1)) + cos(th4)*sin(th1)*sin(th2)) - sin(th6)*(cos(th5)*(cos(th4)*(cos(th1)*sin(th3) + cos(th2)*cos(th3)*sin(th1)) - sin(th1)*sin(th2)*sin(th4)) + sin(th5)*(cos(th1)*cos(th3) - cos(th2)*sin(th1)*sin(th3))), cos(th6)*(cos(th2)*cos(th4) - cos(th3)*sin(th2)*sin(th4)) - sin(th6)*(cos(th5)*(cos(th2)*sin(th4) + cos(th3)*cos(th4)*sin(th2)) - sin(th2)*sin(th3)*sin(th5))];
%%%%%%%%%%%%%%%%%%%%%%%%%%%%%%%%%%%%%%%%%%%%%%%%%%%%
mE=J7*J7t*E;
a = dot(E,mE)/dot(mE,mE);
dQ = a*J7t*E;

%q_new.Position(1) =+ double(dQ(1));
%q_new.Position(2) =+ double(dQ(2));
%q_new.Position(3) =+ double(dQ(3));
%q_new.Position(4) =+ double(dQ(4));
%q_new.Position(5) =+ double(dQ(5));
%q_new.Position(6) =+ double(dQ(6));
%q_new.Position(7) =+ double(dQ(7));

%Z = 0;
%q_new.Position(1) = double(Z);
%q_new.Position(2) = double(Z);
%q_new.Position(3) = double(Z);
%q_new.Position(4) = double(Z);
%q_new.Position(5) = double(Z);
%q_new.Position(6) = double(Z);
%q_new.Position(7) = double(Z);
    
q_new.Header.Seq = uint32(seq);
seq = seq + 1;
end
